simulink model "RC"  (R2021a)
settings: Solver=VariableStepAuto  StartTime=0.0  StopTime=10.0  RelTol=1e-3
values from neighbouring files (symbols this model uses):
  C = input('Enter value of C=')    [RC.m]    (also in RCckt.m = input('C='); tf.m = [1 0])
  R = input('Enter value of R=')    [RC.m]    (also in RCckt.m = input('R='); RLckt.m = input('R='); motor.m)
settings Model: Creator=User  LastModifiedBy=User

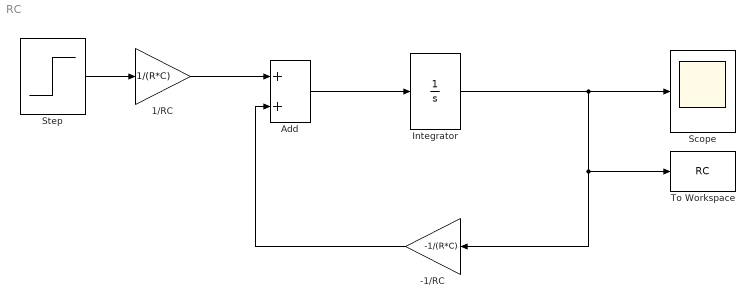
== system RC ==
  -1/RC : Gain  Gain=-1/(R*C)
  1/RC : Gain  Gain=1/(R*C)
  Add : Sum
  Integrator : Integrator
  Scope : Scope
  Step : Step  SampleTime=0
  To Workspace : ToWorkspace  VariableName=RC  SaveFormat=Timeseries  SampleTime=-1
  wires:
  Step/1 -> 1/RC/1
  1/RC/1 -> Add/1
  Add/1 -> Integrator/1
  Integrator/1 -> To Workspace/1, -1/RC/1, Scope/1
  -1/RC/1 -> Add/2
